simulink model "blockResponse"  (R2024a)
settings: Solver=FixedStepAuto  StartTime=0.0  StopTime=simtime  RelTol=1e-9  EnableMultiTasking=on
values from neighbouring files (symbols this model uses):
  consecutive_step_length = 2.5    [writeBlockResponse.m]    (also in writeWResponse.m)
  initial_step_length = 7.5    [writeBlockResponse.m]    (also in writeWResponse.m)
  u_eq = 152    [systemIdentification.m]    (also in writeBlockResponse.m = 151; writeWResponse.m = 152.5)
  u_max = u_maxs(i)    [writeBlockResponse.m]    (also in writeWResponse.m = 170)
  u_step = u_steps(j)    [writeBlockResponse.m]    (also in writeWResponse.m = 8)
undefined symbols (not defined in the file or in its folder): ln
libraries: arduinolib x2
settings Model: ExtModeTrigDuration=2  Creator=twallema  LastModifiedBy=twallema
settings SolverCC: AlgebraicLoopSolver=TrustRegion
settings OptimizationCC: EnhancedBackFolding=on  PassReuseOutputArgsThreshold=0  MaxStackSize=64  OptimizeBlockOrder=speed  DifferentSizesBufferReuse=on  OptimizationCustomize=off
settings DebuggingCC: ParameterTunabilityLossMsg=error  UnconnectedInputMsg=warning  UnconnectedOutputMsg=warning  UnconnectedLineMsg=warning
settings HardwareCC: ProdBitPerInt=16  ProdBitPerPointer=16  ProdBitPerSizeT=16  ProdBitPerPtrDiffT=16  ProdLargestAtomicFloat=None  ProdWordSize=8  ProdHWDeviceType=Atmel->AVR  UseEmbeddedCoderFeatures=off  UseSimulinkCoderFeatures=off
settings ModelReferenceCC: EnableRefExpFcnMdlSchedulingChecks=on
settings SFSimCC: MATLABDynamicMemAlloc=off  CustomCodeUndefinedFunction=UseInterfaceOnly
settings RTWCC: Description=Embedded Coder  SystemTargetFile=ert.tlc  HardwareBoard=Arduino Uno  TemplateMakefile=ert_default_tmf  GenerateReport=on  Toolchain=Arduino AVR  BuildConfiguration=Faster Runs  LaunchReport=on  GPUComputeCapability=3.5  DLArmComputeVersion=19.05
settings CodeAppCC: ForceParamTrailComments=on  OperatorAnnotations=on
settings ERTTargetCC: ERTCustomFileBanners=off  SupportContinuousTime=on  SupportNonInlinedSFcns=on  RemoveResetFunc=off  SupportVariableSizeSignals=on  ModelStepFunctionPrototypeControlCompliant=off  ExtModeStaticAllocSize=250

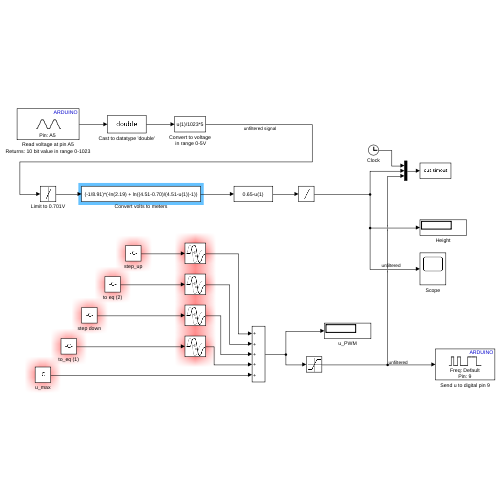
[thumbnail: Simulink's stored preview of the top-level diagram]
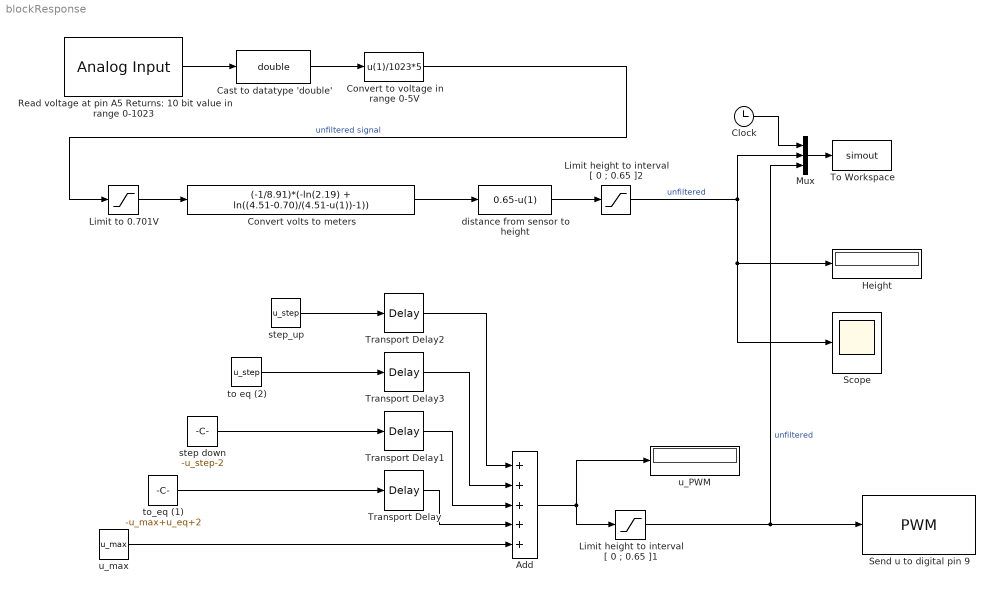
== system blockResponse ==
  Add : Sum  Inputs=+++++
  Cast to datatype 'double' : DataTypeConversion  OutDataTypeStr=double  SaturateOnIntegerOverflow=off  RndMeth=Floor
  Clock : Clock
  Convert to voltage in range 0-5V : Fcn  Expr=u(1)/1023*5
  Convert volts to meters : Fcn  Expr=(-1/8.91)*(-ln(2.19) + ln((4.51-0.70)/(4.51-u(1))-1))
  Height : Display
  Limit height to interval [ 0 ; 0.65 ]1 : Saturate  UpperLimit=255  LowerLimit=0
  Limit height to interval [ 0 ; 0.65 ]2 : Saturate  UpperLimit=0.62  LowerLimit=0
  Limit to 0.701V : Saturate  UpperLimit=inf  LowerLimit=0.701
  Mux : Mux  Inputs=3
  Read voltage at pin A5 Returns: 10 bit value in range 0-1023 : arduinolib/Analog Input  pinNumber=5  ReadResultsOnly=off  ConversionTriggerSource=Software  ExternalTriggerType=uint32(0)  OutputDataType=uint16  EnableConversionCompleteNotify=off  EnableOuputStatus=off  SampleTime=0.05  blockPlatform=arduino
  Scope : Scope
  Send u to digital pin 9 : arduinolib/PWM  pinNumber=9  frequencyType=Default  desiredFrequency=490.2  achievableFrequency=490.2
  To Workspace : ToWorkspace  VariableName=simout  SampleTime=-1
      settings: Save2DSignal=2-D array (concatenate along first dimension)
  Transport Delay : TransportDelay  DelayTime=initial_step_length
  Transport Delay1 : TransportDelay  DelayTime=initial_step_length + 3*consecutive_step_length
  Transport Delay2 : TransportDelay  DelayTime=initial_step_length + 6*consecutive_step_length
  Transport Delay3 : TransportDelay  DelayTime=initial_step_length + 4*consecutive_step_length
  distance from sensor to height : Fcn  Expr=0.65-u(1)
  step down : Constant  Value=-u_step-2  VectorParams1D=off
  step_up : Constant  Value=u_step  VectorParams1D=off
  to eq (2) : Constant  Value=u_step  VectorParams1D=off
  to_eq (1) : Constant  Value=-u_max+u_eq+2  VectorParams1D=off
  u_PWM : Display
  u_max : Constant  Value=u_max
  wires:
  Read voltage at pin A5 Returns: 10 bit value in range 0-1023/1 -> Cast to datatype 'double'/1
  Cast to datatype 'double'/1 -> Convert to voltage in range 0-5V/1
  Clock/1 -> Mux/1
  Limit height to interval [ 0 ; 0.65 ]2/1 -> Mux/2, Height/1, Scope/1  "unfiltered"
  Convert volts to meters/1 -> distance from sensor to height/1
  distance from sensor to height/1 -> Limit height to interval [ 0 ; 0.65 ]2/1
  Limit to 0.701V/1 -> Convert volts to meters/1
  Convert to voltage in range 0-5V/1 -> Limit to 0.701V/1  "unfiltered signal"
  Mux/1 -> To Workspace/1
  to_eq (1)/1 -> Transport Delay/1
  Add/1 -> u_PWM/1, Limit height to interval [ 0 ; 0.65 ]1/1
  Limit height to interval [ 0 ; 0.65 ]1/1 -> Mux/3, Send u to digital pin 9/1  "unfiltered"
  step down/1 -> Transport Delay1/1
  step_up/1 -> Transport Delay2/1
  to eq (2)/1 -> Transport Delay3/1
  Transport Delay3/1 -> Add/2
  u_max/1 -> Add/5
  Transport Delay/1 -> Add/4
  Transport Delay1/1 -> Add/3
  Transport Delay2/1 -> Add/1
